simulink model "CascadeCompositionExample_PedestrianLightwithCarLight"  (R2023a)
settings: Solver=FixedStepAuto  StartTime=0.0  StopTime=300  FixedStep=1  RelTol=1e-3
settings Model: Creator=Administrator  LastModifiedBy=wkmiao
settings RTWCC: GPUComputeCapability=5.0

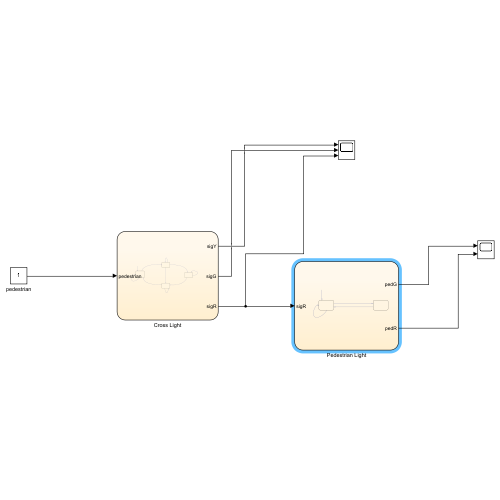
[thumbnail: Simulink's stored preview of the top-level diagram]
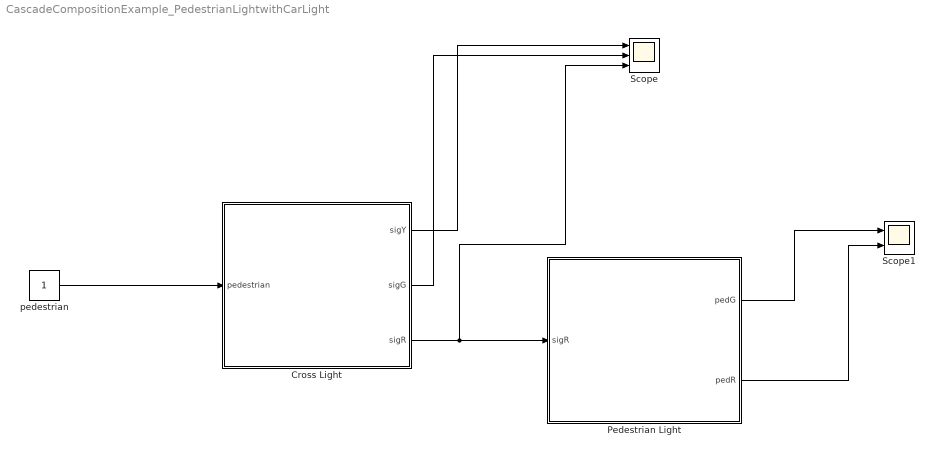
== system CascadeCompositionExample_PedestrianLightwithCarLight ==
  Cross Light : Stateflow chart  TreatAsAtomicUnit=on
  Pedestrian Light : Stateflow chart  TreatAsAtomicUnit=on
  Scope : Scope  NumInputPorts=3
  Scope1 : Scope  NumInputPorts=2
  pedestrian : Constant
  wires:
  Cross Light/3(sigR) -> Scope/3, Pedestrian Light/1(sigR)
  pedestrian/1 -> Cross Light/1(pedestrian)
  Cross Light/1(sigY) -> Scope/1
  Cross Light/2(sigG) -> Scope/2
  Pedestrian Light/1(pedG) -> Scope1/1
  Pedestrian Light/2(pedR) -> Scope1/2

== stateflow chart CascadeCompositionExample_PedestrianLightwithCarLight/Cross Light ==
  state green
  state red
    exit:
    sigR = 0
  state pending
  state yellow
  green -> green [order 3] : [count < 60]{count = count +1}
  red -> green [order 1] : [count >= 60]{sigG = 1;count =0}
  green -> pending [order 1] : [pedestrian & count < 60]{count = count + 1}
  (default) -> red : {count = 0}
  green -> yellow [order 2] : [pedestrian & count >=60]{sigY = 1;count =0}
  pending -> pending [order 2] : {count = count +1}
  red -> red [order 2] : {count = count + 1}
  yellow -> red [order 1] : [count >= 5]{sigR = 1;count =0}
  pending -> yellow [order 1] : [count >= 60]{sigY = 1; count = 0}
  yellow -> yellow [order 2] : {count = count +1}
  data: sigY output; pedestrian input; count local; sigG output; sigR output

== stateflow chart CascadeCompositionExample_PedestrianLightwithCarLight/Pedestrian Light ==
  settings: initializeOutput=1
  state green
  state red
  (default) -> green : {pcount = 0}
  green -> red [order 1] : [pcount >= 55 ]{pedR = 1}
  green -> green [order 2] : {pcount = pcount + 1}
  red -> green : [sigR]{pedG = 1;pcount =0}
  data: sigR input; pcount local; pedG output; pedR output
